simulink model "regulator_calkowanie"  (R2024b)
settings: Solver=VariableStepAuto  StartTime=0.0  StopTime=100  RelTol=1e-3
values from neighbouring files (symbols this model uses):
  y_zad = 5    [wykresy_regulator_calkowy.m]
undefined symbols (not defined in the file or in its folder): K_2, K_I
settings Model: Creator=mparadow  LastModifiedBy=mparadow

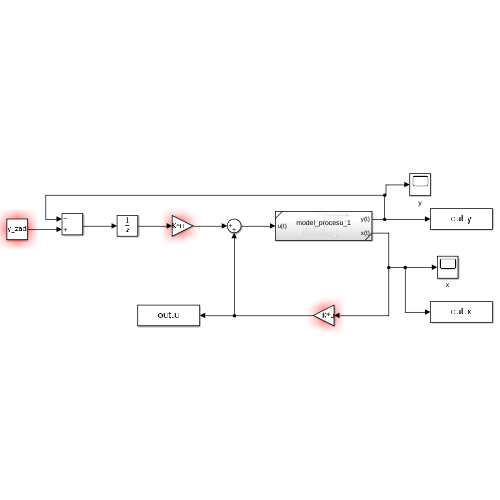
[thumbnail: Simulink's stored preview of the top-level diagram]
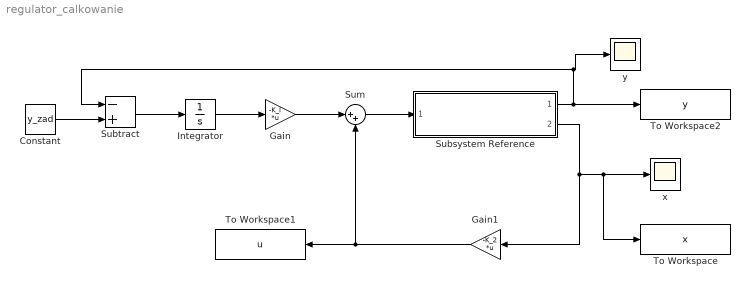
== system regulator_calkowanie ==
  Constant : Constant  Value=y_zad
  Gain : Gain  Gain=-K_I  Multiplication=Matrix(K*u)
  Gain1 : Gain  Gain=-K_2  Multiplication=Matrix(K*u)
  Integrator : Integrator
  Subsystem Reference : Subsystem  ReferencedSubsystem=model_procesu_1
  Subtract : Sum  Inputs=-+
  Sum : Sum  Inputs=|++
  To Workspace : ToWorkspace  VariableName=x  SaveFormat=Structure With Time  SampleTime=-1
  To Workspace1 : ToWorkspace  VariableName=u  SaveFormat=Structure With Time  SampleTime=-1
  To Workspace2 : ToWorkspace  VariableName=y  SaveFormat=Structure With Time  SampleTime=-1
  x : Scope
  y : Scope
  wires:
  Subsystem Reference/2 -> Gain1/1, To Workspace/1, x/1
  Subsystem Reference/1 -> Subtract/1, y/1, To Workspace2/1
  Gain1/1 -> Sum/2, To Workspace1/1
  Sum/1 -> Subsystem Reference/1
  Gain/1 -> Sum/1
  Integrator/1 -> Gain/1
  Subtract/1 -> Integrator/1
  Constant/1 -> Subtract/2
